simulink model "foc_demo"  (R2016b)
settings: Solver=VariableStepAuto  StartTime=0.0  StopTime=10.0  RelTol=1e-6
libraries: powerlib x4, powerlib_meascontrol x3
settings Model: SimulationMode=rapid-accelerator  Creator=USER  LastModifiedBy=USER
settings SolverCC: ZeroCrossAlgorithm=Adaptive

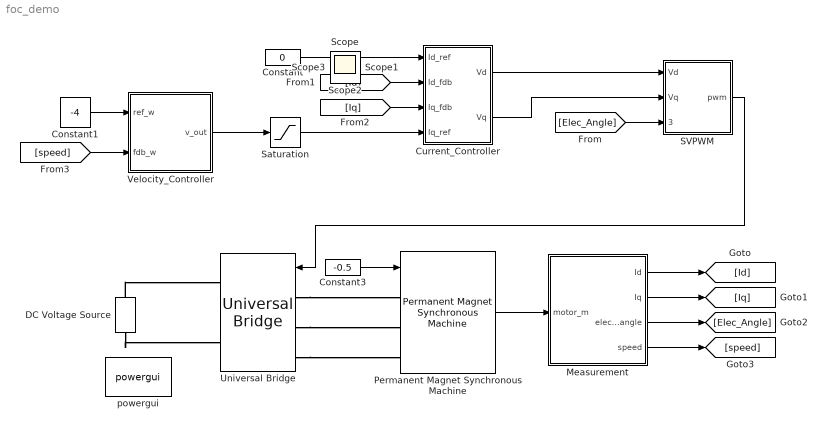
== system foc_demo ==
  Constant : Constant  Value=0
  Constant1 : Constant  Value=-4
  Constant3 : Constant  Value=-0.5
  Current_Controller : Subsystem
  DC Voltage Source : powerlib/Electrical Sources/DC Voltage Source  Amplitude=40  Measurements=None
  Measurement : Subsystem
  Permanent Magnet Synchronous Machine : powerlib/Machines/Permanent Magnet Synchronous Machine  NbPhases=3  FluxDistribution=Sinusoidal  RotorType=Round  MechanicalLoad=Torque Tm  PresetModel=No  ShowDetailedParameters=on  MeasurementBus=off  Resistance=2.85  Inductance=8.5e-3  dqInductances=[8.5e-3,8.5e-3]  La=0.00395  MachineConstant=Torque Constant (N.m / A_peak)  Flux=0.1194  VoltageCst=86.6271  TorqueCst=0.7164  Flat=120  Mechanical=[0.027 0.0004924 4 0]  PolePairs=4  InitialConditions=[0,0, 0,0]  InitialConditions5ph=[0 0 0 0 0 0]  TsPowergui=0  TsBlock=-1  RefAngle=Aligned with phase A axis (original Park)
  SVPWM : Subsystem
  Saturation : Saturate  UpperLimit=3  LowerLimit=-3
  Universal Bridge : powerlib/Power Electronics/Universal Bridge  Arms=3  SnubberResistance=1e5  SnubberCapacitance=inf  Device=IGBT / Diodes  Ron=1e-3  Lon=0  ForwardVoltages="[  0  0  ]"  ForwardVoltage=0  GTOparameters=[ 10e-6 , 20e-6 ]  IGBTparameters=[ 1e-6 , 2e-6 ]  Measurements=All voltages and currents  Measurements_2=None  converterType=Rectifier
  Velocity_Controller : Subsystem  mask{kp=10, ki=10}
      mask prompts: kp "Kp of controller"; ki "Ki of controller"
      settings: AttributesFormatString=|
      | Kp of Controller:%<kp>
      | Ki of Controller:%<ki>
      mask DialogControl DescTextVar Prompt: PI Controller of BLDC speed loop
  powergui : powerlib/powergui  Priority=1  SimulationMode=Continuous  SolverType=Tustin/Backward Euler (TBE)  SampleTime=50e-6  frequency=60  SPID=off  DisableSnubberDevices=off  DisableRonSwitches=off  DisableVfSwitches=off  SwTol=0  DisplayEquations=off  Interpol=off  ExternalGateDelay=off  methode=off  Ts=10  FunctionMessages=off  echomessages=off  HookPort=off  EnableUseOfTLC=off  x0status=blocks  frequencyindice=0  Pbase=100e6  ErrMax=1e-4  Iterations=50  UnitsV=kV  UnitsW=MW  buscounter=0  RestoreLinks=warning  ResistiveCurrentMeasurement=off  Frange=[0:2:500]  Ylog=off  Xlog=on  ShowGrid=off  save=off  variable=ZData  structure=0  ZoomFFT=off  StartTime=0.0  cycles=1  DisplayStyle=1  fundamental=60  FreqAxis=off  MaxFrequency=1000  frequencyindicesteady=1  RmsSteady=1  display=off
  Scope{,1..3} (4 alike) : Scope
  wires:
  Constant3/1 -> Permanent Magnet Synchronous Machine/1
  Permanent Magnet Synchronous Machine/1 -> Measurement/1(motor_m)
  [Elec_Angle] -> SVPWM/3(electrical_angle)
  SVPWM/1(pwm) -> Universal Bridge/1
  Measurement/1(Id) -> [Id]
  Measurement/2(Iq) -> [Iq]
  Measurement/3(electrical_angle) -> [Elec_Angle]
  Measurement/4(speed) -> [speed]
  Velocity_Controller/1(v_out) -> Saturation/1
  Constant1/1 -> Velocity_Controller/1(ref_w)
  [speed] -> Velocity_Controller/2(fdb_w)
  Constant/1 -> Current_Controller/1(Id_ref)
  [Id] -> Current_Controller/2(Id_fdb)
  [Iq] -> Current_Controller/3(Iq_fdb)
  Saturation/1 -> Current_Controller/4(Iq_ref)
  Current_Controller/1(Vd) -> SVPWM/1(Vd)
  Current_Controller/2(Vq) -> SVPWM/2(Vq)
  connections:
  Universal Bridge/LConn1 -- Permanent Magnet Synchronous Machine/LConn1
  Universal Bridge/LConn2 -- Permanent Magnet Synchronous Machine/LConn2
  Universal Bridge/LConn3 -- Permanent Magnet Synchronous Machine/LConn3
  DC Voltage Source/RConn1 -- Universal Bridge/RConn1
  DC Voltage Source/LConn1 -- Universal Bridge/RConn2

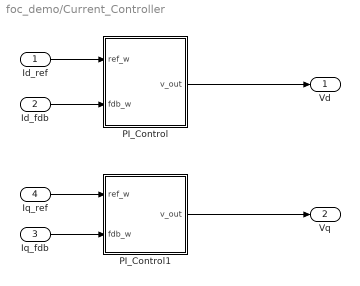
== system foc_demo/Current_Controller ==
  Id_ref : Inport
  Id_fdb : Inport  Port=2
  Iq_fdb : Inport  Port=3
  Iq_ref : Inport  Port=4
  PI_Control : Subsystem  mask{kp=10, ki=1}
      mask prompts: kp "Kp of controller"; ki "Ki of controller"
      settings: AttributesFormatString=|
      | Kp of Controller:%<kp>
      | Ki of Controller:%<ki>
      mask DialogControl DescTextVar Prompt: PI Controller of BLDC speed loop
  PI_Control1 : Subsystem  mask{kp=10, ki=1}
      mask prompts: kp "Kp of controller"; ki "Ki of controller"
      settings: AttributesFormatString=|
      | Kp of Controller:%<kp>
      | Ki of Controller:%<ki>
      mask DialogControl DescTextVar Prompt: PI Controller of BLDC speed loop
  Vd : Outport
  Vq : Outport  Port=2
  wires:
  Id_fdb/1 -> PI_Control/2(fdb_w)
  Iq_fdb/1 -> PI_Control1/2(fdb_w)
  Id_ref/1 -> PI_Control/1(ref_w)
  Iq_ref/1 -> PI_Control1/1(ref_w)
  PI_Control1/1(v_out) -> Vq/1
  PI_Control/1(v_out) -> Vd/1

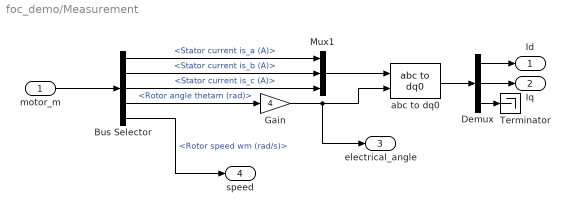
== system foc_demo/Measurement ==
  motor_m : Inport
  Bus Selector : BusSelector  OutputSignals=Stator current is_a (A),Stator current is_b (A),Stator current is_c (A),Rotor angle thetam (rad),Rotor speed wm (rad/s)
  Demux : Demux  Outputs=3
  Gain : Gain  Gain=4
  Mux1 : Mux  Inputs=3
  Terminator : Terminator
  abc to dq0 : powerlib_meascontrol/Transformations/abc to dq0  Alignment=Aligned with phase A axis
  Id : Outport
  Iq : Outport  Port=2
  electrical_angle : Outport  Port=3
  speed : Outport  Port=4
  wires:
  motor_m/1 -> Bus Selector/1
  Bus Selector/1 -> Mux1/1  "<Stator current is_a (A)>"
  Bus Selector/2 -> Mux1/2  "<Stator current is_b (A)>"
  Bus Selector/3 -> Mux1/3  "<Stator current is_c (A)>"
  Mux1/1 -> abc to dq0/1
  abc to dq0/1 -> Demux/1
  Bus Selector/4 -> Gain/1  "<Rotor angle thetam (rad)>"
  Bus Selector/5 -> speed/1  "<Rotor speed wm (rad/s)>"
  Demux/1 -> Id/1
  Demux/2 -> Iq/1
  Demux/3 -> Terminator/1
  Gain/1 -> electrical_angle/1, abc to dq0/2

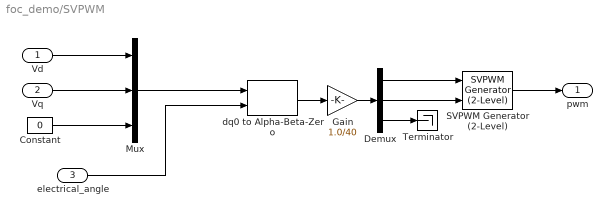
== system foc_demo/SVPWM ==
  Vd : Inport
  Vq : Inport  Port=2
  electrical_angle : Inport  Port=3
  Constant : Constant  Value=0
  Demux : Demux  Outputs=3
  Gain : Gain  Gain=1.0/40
  Mux : Mux  Inputs=3
  SVPWM Generator (2-Level) : powerlib_meascontrol/Pulse & Signal Generators/SVPWM Generator (2-Level)  InputType=alpha-beta components  SwitchingPattern=Pattern #1  Fc=5000  ParUref=[0.8 -30 50]  Ts=0
  Terminator : Terminator
  dq0 to Alpha-Beta-Zero : powerlib_meascontrol/Transformations/dq0 to Alpha-Beta-Zero  Alignment=Aligned with phase A axis
  pwm : Outport
  wires:
  SVPWM Generator (2-Level)/1 -> pwm/1
  Demux/2 -> SVPWM Generator (2-Level)/2
  Demux/3 -> Terminator/1
  Demux/1 -> SVPWM Generator (2-Level)/1
  dq0 to Alpha-Beta-Zero/1 -> Gain/1
  Mux/1 -> dq0 to Alpha-Beta-Zero/1
  Vq/1 -> Mux/2
  Vd/1 -> Mux/1
  Constant/1 -> Mux/3
  electrical_angle/1 -> dq0 to Alpha-Beta-Zero/2
  Gain/1 -> Demux/1

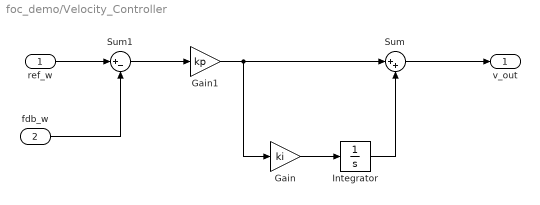
== system foc_demo/Velocity_Controller ==
  ref_w : Inport
  fdb_w : Inport  Port=2
  Gain : Gain  Gain=ki
  Gain1 : Gain  Gain=kp
  Integrator : Integrator
  Sum : Sum  Inputs=|++
  Sum1 : Sum  Inputs=|+-
  v_out : Outport
  wires:
  fdb_w/1 -> Sum1/2
  Sum/1 -> v_out/1
  Sum1/1 -> Gain1/1
  Integrator/1 -> Sum/2
  ref_w/1 -> Sum1/1
  Gain/1 -> Integrator/1
  Gain1/1 -> Gain/1, Sum/1

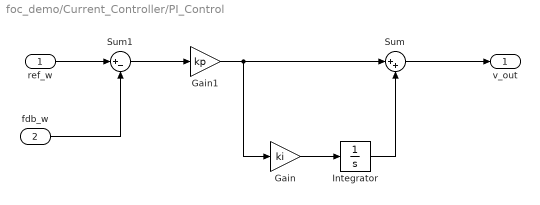
== system foc_demo/Current_Controller/PI_Control ==
  ref_w : Inport
  fdb_w : Inport  Port=2
  Gain : Gain  Gain=ki
  Gain1 : Gain  Gain=kp
  Integrator : Integrator
  Sum : Sum  Inputs=|++
  Sum1 : Sum  Inputs=|+-
  v_out : Outport
  wires:
  fdb_w/1 -> Sum1/2
  Sum/1 -> v_out/1
  Sum1/1 -> Gain1/1
  Integrator/1 -> Sum/2
  ref_w/1 -> Sum1/1
  Gain/1 -> Integrator/1
  Gain1/1 -> Gain/1, Sum/1

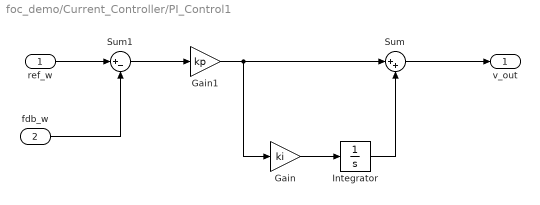
== system foc_demo/Current_Controller/PI_Control1 ==
  ref_w : Inport
  fdb_w : Inport  Port=2
  Gain : Gain  Gain=ki
  Gain1 : Gain  Gain=kp
  Integrator : Integrator
  Sum : Sum  Inputs=|++
  Sum1 : Sum  Inputs=|+-
  v_out : Outport
  wires:
  fdb_w/1 -> Sum1/2
  Sum/1 -> v_out/1
  Sum1/1 -> Gain1/1
  Integrator/1 -> Sum/2
  ref_w/1 -> Sum1/1
  Gain/1 -> Integrator/1
  Gain1/1 -> Gain/1, Sum/1
